simulink model "robot_echant_etu2"  (R2020b)
settings: Solver=VariableStepAuto  StartTime=0.0  StopTime=10.0  RelTol=1e-3
values from neighbouring files (symbols this model uses):
  delta_t = 0.001    [simu_robot_etu.m]
  K = -place(A,B,V)    [matrices.m]    (also in simu_robot_etu.m = [0.6700   19.9055    1.0747    1.9614])
  ue = 0    [simu_robot_etu.m]
  x0 = [0 pi/10 0 0]    [simu_robot_etu.m]
  xe = [0 0 0 0]'    [simu_robot_etu.m]
undefined symbols (not defined in the file or in its folder): DiscIntNeverNeededParam
libraries: simulink x1
settings Model: Creator=cdelmair  LastModifiedBy=pgonthie
settings DebuggingCC: SFMachineParentedDataDiag=error

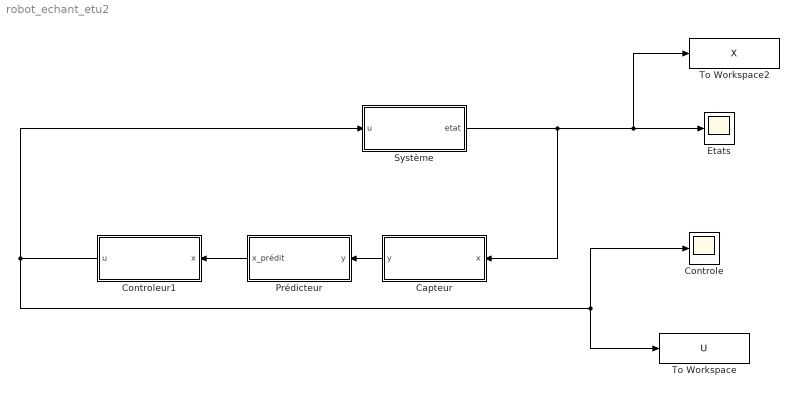
== system robot_echant_etu2 ==
  Capteur : Subsystem
  Controle : Scope
  Controleur1 : Subsystem
  Etats : Scope
  Prédicteur : Subsystem
  Système : Subsystem
  To Workspace : ToWorkspace  VariableName=U  SaveFormat=Timeseries  SampleTime=-1
  To Workspace2 : ToWorkspace  VariableName=X  SaveFormat=Timeseries  SampleTime=-1
  wires:
  Controleur1/1(u) -> To Workspace/1, Controle/1, Système/1(u)
  Système/1(etat) -> To Workspace2/1, Etats/1, Capteur/1(x)
  Prédicteur/1(x_prédit) -> Controleur1/1(x)
  Capteur/1(y) -> Prédicteur/1(y)

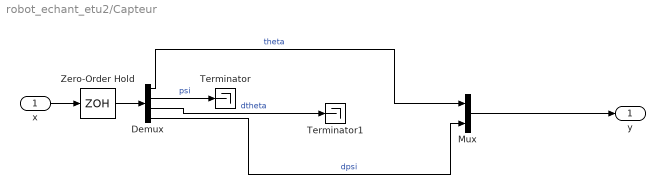
== system robot_echant_etu2/Capteur ==
  x : Inport
  Demux : Demux
  Mux : Mux  Inputs=2
  Terminator : Terminator
  Terminator1 : Terminator
  Zero-Order Hold : ZeroOrderHold  SampleTime=delta_t
  y : Outport
  wires:
  Demux/1 -> Mux/1  "theta"
  Demux/4 -> Mux/2  "dpsi"
  Demux/2 -> Terminator/1  "psi"
  Demux/3 -> Terminator1/1  "dtheta"
  Mux/1 -> y/1
  x/1 -> Zero-Order Hold/1
  Zero-Order Hold/1 -> Demux/1

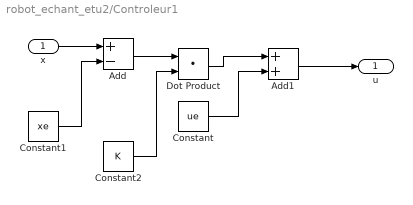
== system robot_echant_etu2/Controleur1 ==
  x : Inport
  Add : Sum  Inputs=+-
  Add1 : Sum
  Constant : Constant  Value=ue
  Constant1 : Constant  Value=xe
  Constant2 : Constant  Value=K
  Dot Product : DotProduct  InputSameDT=on  OutDataTypeStr=Inherit: Inherit via internal rule
  u : Outport
  wires:
  x/1 -> Add/1
  Constant1/1 -> Add/2
  Constant/1 -> Add1/2
  Add1/1 -> u/1
  Dot Product/1 -> Add1/1
  Add/1 -> Dot Product/1
  Constant2/1 -> Dot Product/2

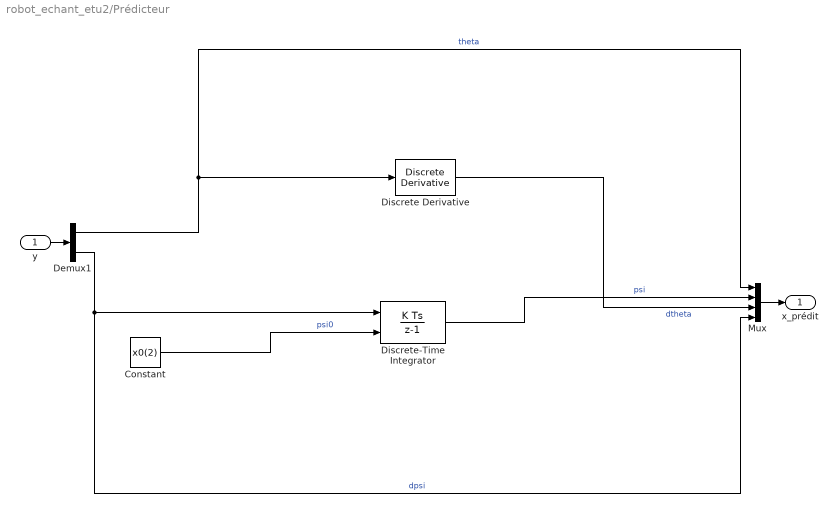
== system robot_echant_etu2/Prédicteur ==
  y : Inport
  Constant : Constant  Value=x0(2)
  Demux1 : Demux  Outputs=2
  Discrete Derivative : simulink/Discrete/Discrete Derivative  gainval=1.0  ICPrevScaledInput=0.0  OutMin=[]  OutMax=[]  OutDataType=fixdt(1, 16)  OutScaling=2^-10  DoSatur=off
  Discrete-Time Integrator : DiscreteIntegrator  InitialConditionSource=external  SampleTime=delta_t  ICPrevOutput=DiscIntNeverNeededParam  ICPrevScaledInput=DiscIntNeverNeededParam
  Mux : Mux
  x_prédit : Outport
  wires:
  Mux/1 -> x_prédit/1
  y/1 -> Demux1/1
  Demux1/1 -> Discrete Derivative/1, Mux/1  "theta"
  Demux1/2 -> Discrete-Time Integrator/1, Mux/4  "dpsi"
  Discrete Derivative/1 -> Mux/3  "dtheta"
  Discrete-Time Integrator/1 -> Mux/2  "psi"
  Constant/1 -> Discrete-Time Integrator/2  "psi0"

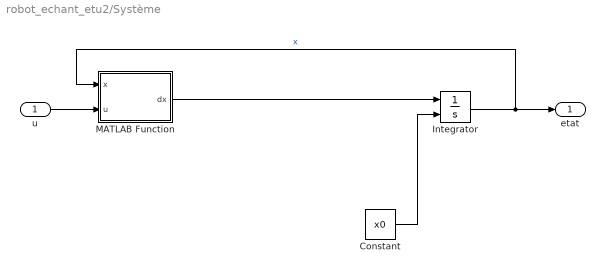
== system robot_echant_etu2/Système ==
  u : Inport
  Constant : Constant  Value=x0
  Integrator : Integrator  InitialConditionSource=external
  MATLAB Function : MATLAB Function  TreatAsAtomicUnit=on
  etat : Outport
  wires:
  Integrator/1 -> etat/1, MATLAB Function/1(x)  "x"
  Constant/1 -> Integrator/2
  u/1 -> MATLAB Function/2(u)
  MATLAB Function/1(dx) -> Integrator/1

== matlab function robot_echant_etu2/Système/MATLAB Function ==
  data: x input; u input; dx output
function dx   = fonction( x, u)
%   Dynamic equations of motion of the segway on an axis.
%   Inputs: - x = [theta psi dtheta dpsi]
%               theta: average angle of the wheels      [rad]
%               psi: body pitch angle                   [rad]
%               dtheta: average velocity of the wheels  [rad/s]
%               dpsi: body pitch velocity               [rad/s]
%          - u: DC motor voltage (same value for both motors) [V]

    % State
    psi = x(2);
    dtheta = x(3);
    dpsi = x(4);

    % Parameters
    
    g = 9.81;           % gravity acceleration [m/sec^2]
    m = 0.03;           % wheel weight [kg]
    R = 0.04;           % wheel radius [m]
    Jw = m*R^2/2;       % wheel inertia moment [kg*m^2]
    M = 0.6;            % body weight [kg]
    H = 0.144;          % body height [m]
    L = H/2;            % distance of the center of mass from the wheel axle [m]
    Jpsi = M*L^2/3;     % body pitch inertia [kgm^2]
    Jm = 1e-5;          % DC motor inertia moment [kgm^2]
    Rm = 6.69;          % DC motor resistance [Ohm]
    Kb = 0.468;         % DC motor back EMF constant [Vsec/rad]
    Kt = 0.317;         % DC motor torque constant [Nm/A]
    n = 1;              % gear ratio
    fm = 0.0022;        % friction coefficient between body and DC motor
    fw = 0;             % friction coefficient between wheel and floor
    
    % Equations of motion
    c1 = (2*m+M)*R^2 + 2*Jw + 2*n^2*Jm;
    c2 = M*L*R*cos(psi) - 2*n^2*Jm;
    c3 = -M*L*R*dpsi^2*sin(psi);
    c4 = M*L^2 + Jpsi + 2*n^2*Jm;
    c5 = -M*g*L*sin(psi);

    alpha = Kt/Rm;
    beta = Kt*Kb/Rm + fm;

    Ftheta = alpha*(2*u) - 2*(beta+fw)*dtheta + 2*beta*dpsi;
    Fpsi = -alpha*(2*u) + 2*beta*dtheta - 2*beta*dpsi;

    ddtheta = (c4*c3 - c2*c5 + c4*Ftheta - c2*Fpsi)/(c4*c1 - c2^2);
    ddpsi = (Fpsi- c2*ddtheta - c5)/c4;
    dx = [dtheta dpsi ddtheta ddpsi]';

end
